simulink model "No_linear_model"  (R2018a)
settings: Solver=VariableStepAuto  StartTime=0.0  StopTime=100  RelTol=1e-3
values from neighbouring files (symbols this model uses):
  G = 9.81    [Dados.m]    (also in Dados_correct.m)
  L1 = 0.3    [Dados.m]    (also in Dados_correct.m = 0.227; Function_ARE.m = 0.227; areklmn_reactor.m = 0.227; fd0.m = 0.227)
  L2 = 0.1    [Dados.m]    (also in Dados_correct.m = 0.08; Function_ARE.m = 0.08; areklmn_reactor.m = 0.08; fd0.m = 0.08)
  M1 = 0.04    [Dados.m]    (also in Dados_correct.m = 0.2)
  M2 = 0.04    [Dados.m]    (also in Dados_correct.m = 0.2)
settings Model: Creator=stayn  LastModifiedBy=stayn

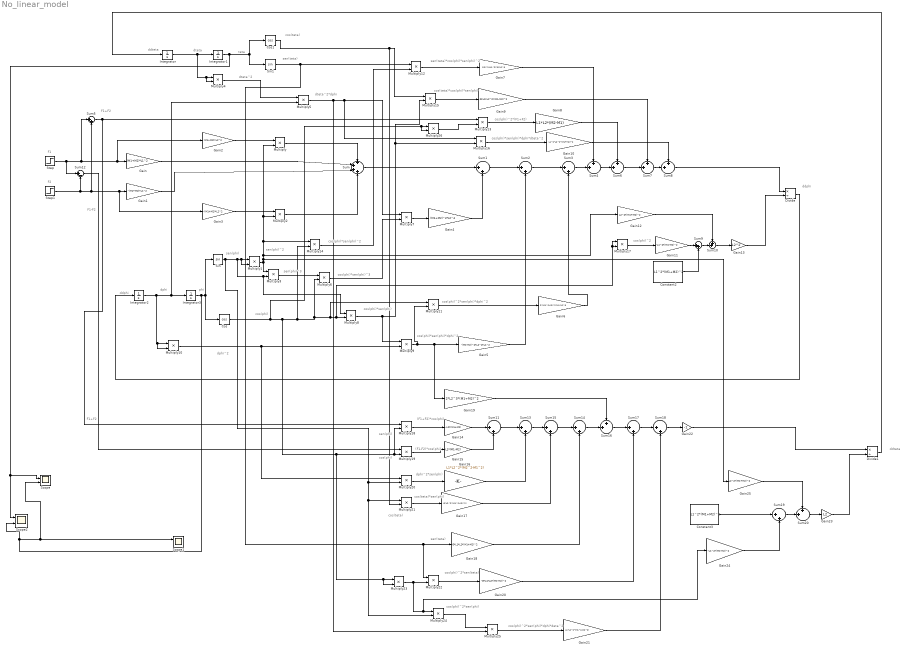
== system No_linear_model ==
  note: ddteta
  note: ddteta
  note: cos(phi)^2*sen(phi)
  note: cos(phi)^2*sen(teta)
  note: cos(phi)
  note: sen(teta)
  note: cos(teta)*sen(phi)
  note: sen(phi)
  note: cos(teta)
  note: dphi^2*sen(phi)
  note: F1-F2
  note: (F1+F2)*cos(phi)
  note: ddphi
  note: ddphi
  note: cos(phi)^2
  note: cos(teta)
  note: cos(phi)^2*(F1+F2)
  note: F1+F2
  note: sen(teta)*cos(phi)*sen(phi)^2
  note: sen(teta)
  note: dphi^2
  note: cos(phi)*sen(phi)*dphi^2
  note: cos(phi)*sen(phi)
  note: cos(phi)*sen(phi)^3
  note: cos(phi)
  note: dteta^2*dphi
  note: dteta^2
  note: sen(phi)
  note: phi
  note: dphi
  note: teta
  note: dteta
  note: F1
  note: F2
  note: sen(phi)^2
  note: sen(phi)^3
  note: cos(phi)^2*sen(phi)*dphi^2
  note: cos(phi)*sen(phi)^2
  note: cos(teta)*cos(phi)*sen(phi)
  note: cos(phi)*sen(phi)*dphi*dteta^2
  note: F1+F2
  note: (F1-F2)*cos(phi)
  note: cos(phi)^2*sen(phi)*dphi*deta^2
  Constant2 : Constant  Value=L1^2*(M1+M2)^2
  Constant3 : Constant  Value=L1^2*(M1+M2)^2
  Cos : Trigonometry  Operator=cos
  Cos1 : Trigonometry  Operator=cos
  Divide : Product  Inputs=*/
  Divide1 : Product  Inputs=*/
  Gain : Gain  Gain=(M1+M2)*L1^2
  Gain1 : Gain  Gain=-(M1+M2)*L1^2
  Gain10 : Gain  Gain=L1^2*L2^2*(M1+M2)^2
  Gain11 : Gain  Gain=-L1^2*(M1-M2)^2
  Gain12 : Gain  Gain=L2^2*(M1+M2)^2
  Gain13 : Gain  Gain=L2^2
  Gain14 : Gain  Gain=-L2*(M1+M2)
  Gain15 : Gain  Gain=L1*(M1-M2)
  Gain16 : Gain  Gain=L1*L2^2*(M2^2-M1^2)
  Gain17 : Gain  Gain=G*L2^2*(M1^2-M2^2)
  Gain18 : Gain  Gain=G*L1*L2*(M1+M2)^2
  Gain19 : Gain  Gain=2*L2^3*(M1+M2)^2
  Gain2 : Gain  Gain=(M1+M2)*L2^2
  Gain20 : Gain  Gain=-G*L1*L2*(M1-M2)^2
  Gain21 : Gain  Gain=L1*L2^2*(M1^2-M2^2)
  Gain22 : Gain  Gain=-1
  Gain23 : Gain  Gain=L2
  Gain24 : Gain  Gain=-L1^2*(M1-M2)^2
  Gain25 : Gain  Gain=L2^2*(M1+M2)^2
  Gain3 : Gain  Gain=-(M1+M2)*L2^2
  Gain4 : Gain  Gain=(M1+M2)^2*L2^4
  Gain5 : Gain  Gain=-(M1-M2)^2*L2^2*L1^2
  Gain6 : Gain  Gain=2*(M1^2-M2^2)*L1*L2^3
  Gain7 : Gain  Gain=(M2^2-M1^2)*G*L2^3
  Gain8 : Gain  Gain=L1*L2*(M2-M1)
  Gain9 : Gain  Gain=G*L1*L2^2*(M1-M2)^2
  Integrator{,1..3} (4 alike) : Integrator
  Multiply{,1..26} (27 alike) : Product
  Scope : Scope  NumInputPorts=2
  Scope1 : Scope  NumInputPorts=2
  Scope2 : Scope  NumInputPorts=2
  Sin : Trigonometry
  Sin1 : Trigonometry
  Step : Step  After=0.005  SampleTime=0
  Step1 : Step  After=0.005  SampleTime=0
  Sum : Sum  Inputs=++++
  Sum{1..3,5,9,11,13..15,17..19} (12 alike) : Sum  Inputs=|++
  Sum{4,6..8,10,16,20} (7 alike) : Sum  Inputs=++|
  Sum12 : Sum  Inputs=|+-
  wires:
  Step/1 -> Sum12/1, Sum5/1, Gain2/1, Gain/1
  Gain/1 -> Sum/2
  Gain1/1 -> Sum/3
  Integrator/1 -> Multiply4/2, Multiply4/1, Integrator1/1
  Divide1/1 -> Integrator/1
  Integrator2/1 -> Multiply10/2, Multiply10/1, Multiply5/2, Integrator3/1
  Gain2/1 -> Multiply/1
  Integrator3/1 -> Scope2/2, Scope/2, Scope1/1, Cos/1, Sin/1
  Sin/1 -> Multiply24/2, Multiply21/1, Multiply20/2, Multiply8/1, Multiply3/2, Multiply1/2, Multiply1/1
  Multiply/1 -> Sum/1
  Gain3/1 -> Multiply2/1
  Multiply2/1 -> Sum/4
  Multiply3/1 -> Multiply6/1
  Multiply4/1 -> Multiply5/1
  Multiply5/1 -> Multiply25/2, Multiply16/1, Multiply7/1
  Multiply6/1 -> Multiply7/2
  Sum/1 -> Sum1/1
  Multiply7/1 -> Gain4/1
  Gain4/1 -> Sum1/2
  Multiply9/1 -> Multiply11/2, Gain19/1, Gain5/1
  Gain5/1 -> Sum2/2
  Sum1/1 -> Sum2/1
  Cos/1 -> Multiply26/2, Multiply26/1, Multiply23/2, Multiply23/1, Multiply18/2, Multiply19/2, Multiply14/2, Multiply6/2, Multiply11/1, Multiply17/2, Multiply17/1, Multiply8/2
  Multiply11/1 -> Gain6/1
  Gain6/1 -> Sum3/2
  Sum2/1 -> Sum3/1
  Sin1/1 -> Multiply22/1, Gain18/1, Multiply12/1
  Multiply8/1 -> Multiply16/2, Multiply15/2, Multiply9/1
  Multiply14/1 -> Multiply12/2
  Multiply12/1 -> Gain7/1
  Sum3/1 -> Sum4/2
  Gain7/1 -> Sum4/1
  Sum5/1 -> Multiply18/1, Multiply13/1
  Multiply13/1 -> Gain8/1
  Sum4/1 -> Sum6/2
  Gain8/1 -> Sum6/1
  Cos1/1 -> Multiply15/1, Multiply21/2
  Multiply15/1 -> Gain9/1
  Sum6/1 -> Sum7/2
  Gain9/1 -> Sum7/1
  Sum7/1 -> Sum8/2
  Multiply16/1 -> Gain10/1
  Gain10/1 -> Sum8/1
  Multiply17/1 -> Gain11/1
  Gain11/1 -> Sum9/1
  Constant2/1 -> Sum9/2
  Sum9/1 -> Sum10/2
  Gain12/1 -> Sum10/1
  Sum10/1 -> Gain13/1
  Sum8/1 -> Divide/1
  Gain13/1 -> Divide/2
  Divide/1 -> Integrator2/1
  Multiply18/1 -> Gain14/1
  Gain14/1 -> Sum11/1
  Step1/1 -> Sum12/2, Gain3/1, Gain1/1, Sum5/2
  Sum12/1 -> Multiply19/1
  Multiply19/1 -> Gain15/1
  Gain15/1 -> Sum11/2
  Multiply10/1 -> Multiply20/1, Multiply9/2
  Multiply20/1 -> Gain16/1
  Sum11/1 -> Sum13/1
  Gain16/1 -> Sum13/2
  Multiply21/1 -> Gain17/1
  Sum13/1 -> Sum15/1
  Gain17/1 -> Sum15/2
  Sum15/1 -> Sum14/1
  Gain18/1 -> Sum14/2
  Sum14/1 -> Sum16/2
  Gain19/1 -> Sum16/1
  Multiply23/1 -> Gain24/1, Multiply24/1, Multiply22/2
  Multiply22/1 -> Gain20/1
  Sum16/1 -> Sum17/1
  Gain20/1 -> Sum17/2
  Multiply24/1 -> Multiply25/1
  Multiply25/1 -> Gain21/1
  Sum17/1 -> Sum18/1
  Gain21/1 -> Sum18/2
  Sum18/1 -> Gain22/1
  Gain24/1 -> Sum19/2
  Constant3/1 -> Sum19/1
  Multiply1/1 -> Multiply3/1, Gain25/1, Multiply14/1, Multiply/2, Multiply2/2, Gain12/1
  Gain25/1 -> Sum20/1
  Sum19/1 -> Sum20/2
  Sum20/1 -> Gain23/1
  Gain22/1 -> Divide1/1
  Gain23/1 -> Divide1/2
  Integrator1/1 -> Scope2/1, Scope/1, Cos1/1, Sin1/1
  Multiply26/1 -> Multiply13/2
